simulink model "Battery"  (R2020a)
settings: Solver=FixedStepAuto  StartTime=0.0  StopTime=300  FixedStep=1e-5  RelTol=1e-3
InitFcn:
  | init;
values from neighbouring files (symbols this model uses):
  A = diag(Adiag)    [init.m]
  B = B/Cn    [init.m]
  C = eye(n)    [init.m]
  D = zeros(n,1)    [init.m]
  FCC = FCC_Ah*60*60    (= 14400)    [init.m]
  n = 4    [init.m]
  OCV = [2.8 3.4 3.6 3.7 3.8 3.9 4.0 4.1 4.2  4.4   4.6]    [init.m]
  R0 = 1.90e-3    (= 0.0019)    [init.m]
  SOC = [0    0.1    0.2  0.3 0.4   0.5   0.6  0.7  0.8    0.9 1]    [init.m]
  Ts = 0.01    [init.m]
libraries: simulink x3
settings Model: Creator=seeke  LastModifiedBy=seeke

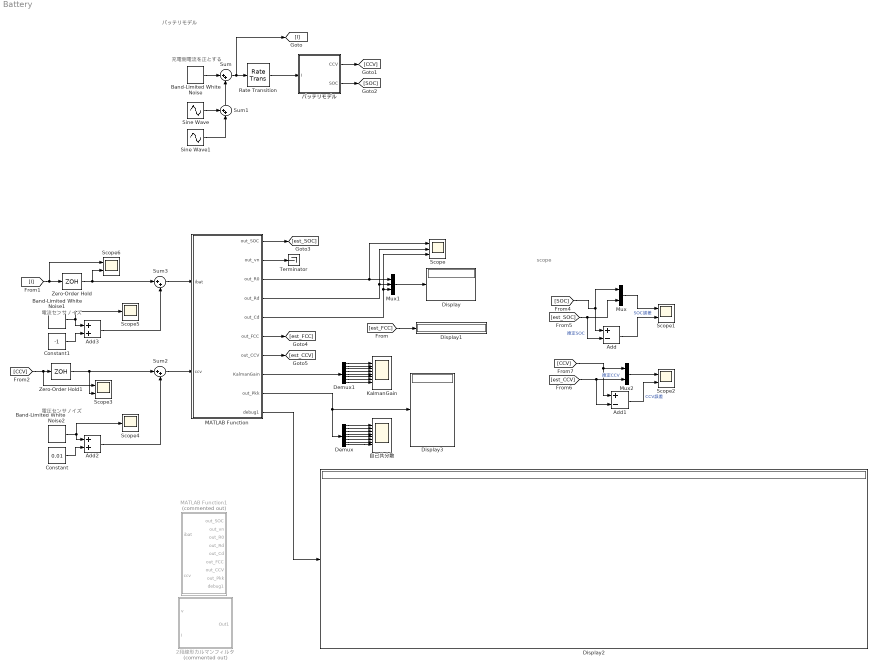
== system Battery ==
  note: 電圧センサノイズ
  note: scope
  note: バッテリモデル
  note: 充電側電流を正とする
  note: 電流センサノイズ
  2段線形カルマンフィルタ : Subsystem  Commented=on
  Add : Sum  Inputs=+-
  Add1 : Sum  Inputs=+-
  Add2 : Sum
  Add3 : Sum
  Band-Limited White Noise : simulink/Sources/Band-Limited White Noise  Cov=[100]  Ts=0.1  seed=[23341]
  Band-Limited White Noise1 : simulink/Sources/Band-Limited White Noise  Cov=[0.01]  Ts=Ts  seed=[6517]
  Band-Limited White Noise2 : simulink/Sources/Band-Limited White Noise  Cov=[0.00003]  Ts=Ts  seed=[50]
  Constant : Constant  Value=0.01
  Constant1 : Constant  Value=-1
  Demux : Demux  Outputs=8
  Demux1 : Demux  Outputs=8
  Display{,1..3} (4 alike) : Display
      Display settings: Format=short_e
      Display1 settings: Format=long_e
      Display2 settings: Format=short_e
      Display3 settings: Format=short_e
  KalmanGain : Scope  NumInputPorts=8
  MATLAB Function : MATLAB Function  TreatAsAtomicUnit=on
  MATLAB Function1 : MATLAB Function  Commented=on  TreatAsAtomicUnit=on
  Mux : Mux  Inputs=2
  Mux1 : Mux  Inputs=3
  Mux2 : Mux  Inputs=2
  Rate Transition : RateTransition
  Scope : Scope  NumInputPorts=3
  Scope{1..3,6} (4 alike) : Scope  NumInputPorts=2
  Scope4 : Scope
  Scope5 : Scope
  Sine Wave : Sin  Amplitude=100  Frequency=2*pi*0.1  SampleTime=0
  Sine Wave1 : Sin  Amplitude=30  Frequency=2*pi*0.01  SampleTime=0
  Sum : Sum  Inputs=|++
  Sum1 : Sum  Inputs=++|
  Sum2 : Sum  Inputs=|++
  Sum3 : Sum  Inputs=|++
  Terminator : Terminator
  Zero-Order Hold : ZeroOrderHold  SampleTime=Ts
  Zero-Order Hold1 : ZeroOrderHold  SampleTime=Ts
  バッテリモデル : Subsystem
  自己共分散 : Scope  NumInputPorts=8
  wires:
  Rate Transition/1 -> バッテリモデル/1(I)
  Sum/1 -> [I], Rate Transition/1
  Band-Limited White Noise/1 -> Sum/1
  バッテリモデル/1(CCV) -> [CCV]
  [CCV] -> Scope3/1, Zero-Order Hold1/1
  Zero-Order Hold1/1 -> Scope3/2, Sum2/1
  [I] -> Scope6/1, Zero-Order Hold/1
  Zero-Order Hold/1 -> Sum3/1, Scope6/2
  バッテリモデル/2(SOC) -> [SOC]
  [SOC] -> Mux/1, Add/1
  MATLAB Function/1(out_SOC) -> [est_SOC]
  MATLAB Function/6(out_FCC) -> [est_FCC]
  MATLAB Function/7(out_CCV) -> [est_CCV]
  [est_SOC] -> Mux/2, Add/2  "推定SOC"
  [CCV] -> Mux2/1, Add1/1
  [est_CCV] -> Mux2/2, Add1/2  "推定CCV"
  Add/1 -> Scope1/2  "SOC誤差"
  Mux/1 -> Scope1/1
  MATLAB Function/4(out_Rd) -> Scope/2, Mux1/2
  Mux1/1 -> Display/1
  MATLAB Function/3(out_R0) -> Scope/1, Mux1/1
  MATLAB Function/5(out_Cd) -> Scope/3, Mux1/3
  [est_FCC] -> Display1/1
  Sine Wave1/1 -> Sum1/2
  Sine Wave/1 -> Sum1/1
  Sum1/1 -> Sum/2
  MATLAB Function/10(debug1) -> Display2/1
  Mux2/1 -> Scope2/1
  Add1/1 -> Scope2/2  "CCV誤差"
  MATLAB Function/9(out_Pkk) -> Demux/1, Display3/1
  Sum2/1 -> MATLAB Function/2(ccv)
  Sum3/1 -> MATLAB Function/1(ibat)
  Add2/1 -> Sum2/2
  Constant/1 -> Add2/2
  MATLAB Function/2(out_vn) -> Terminator/1
  Constant1/1 -> Add3/2
  Add3/1 -> Sum3/2
  Band-Limited White Noise1/1 -> Scope5/1, Add3/1
  Band-Limited White Noise2/1 -> Add2/1, Scope4/1
  Demux/1 -> 自己共分散/1
  Demux/2 -> 自己共分散/2
  Demux/3 -> 自己共分散/3
  Demux/4 -> 自己共分散/4
  Demux/5 -> 自己共分散/5
  Demux/6 -> 自己共分散/6
  Demux/7 -> 自己共分散/7
  Demux/8 -> 自己共分散/8
  Demux1/8 -> KalmanGain/8
  Demux1/3 -> KalmanGain/3
  Demux1/2 -> KalmanGain/2
  Demux1/4 -> KalmanGain/4
  Demux1/7 -> KalmanGain/7
  Demux1/5 -> KalmanGain/5
  Demux1/1 -> KalmanGain/1
  MATLAB Function/8(KalmanGain) -> Demux1/1
  Demux1/6 -> KalmanGain/6

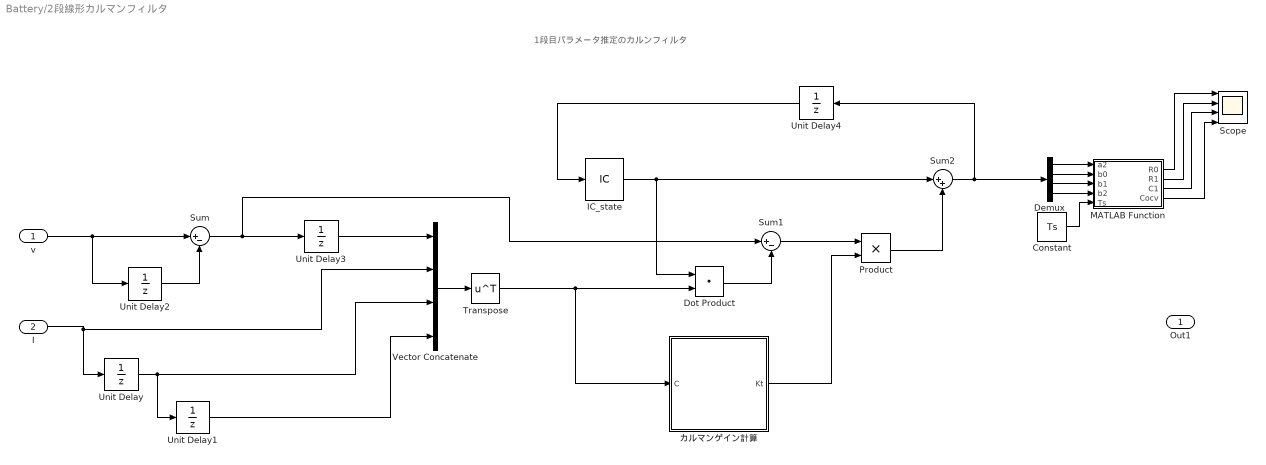
== system Battery/2段線形カルマンフィルタ ==
  note: 1段目パラメータ推定のカルンフィルタ
  v : Inport
  I : Inport  Port=2
  Constant : Constant  Value=Ts
  Demux : Demux
  Dot Product : DotProduct  InputSameDT=on  OutDataTypeStr=Inherit: Inherit via internal rule
  IC_state : InitialCondition  Value=[1 1 1 1]
  MATLAB Function : MATLAB Function  TreatAsAtomicUnit=on
  Product : Product
  Scope : Scope  NumInputPorts=4
  Sum : Sum  Inputs=|+-
  Sum1 : Sum  Inputs=|+-
  Sum2 : Sum  Inputs=|++
  Transpose : Math  Operator=transpose  SaturateOnIntegerOverflow=on
  Unit Delay{,1..4} (5 alike) : UnitDelay  SampleTime=-1  HasFrameUpgradeWarning=on
  Vector Concatenate : Concatenate  NumInputs=4  Mode=Multidimensional array
  カルマンゲイン計算 : MATLAB Function  TreatAsAtomicUnit=on
  Out1 : Outport
  wires:
  Unit Delay/1 -> Vector Concatenate/3, Unit Delay1/1
  I/1 -> Unit Delay/1, Vector Concatenate/2
  Unit Delay1/1 -> Vector Concatenate/4
  v/1 -> Unit Delay2/1, Sum/1
  Unit Delay2/1 -> Sum/2
  Sum/1 -> Sum1/1, Unit Delay3/1
  Unit Delay3/1 -> Vector Concatenate/1
  Vector Concatenate/1 -> Transpose/1
  Dot Product/1 -> Sum1/2
  Sum1/1 -> Product/1
  Product/1 -> Sum2/2
  IC_state/1 -> Sum2/1, Dot Product/1
  Transpose/1 -> Dot Product/2, カルマンゲイン計算/1(C)
  カルマンゲイン計算/1(Kt) -> Product/2
  Unit Delay4/1 -> IC_state/1
  Sum2/1 -> Unit Delay4/1, Demux/1
  Demux/1 -> MATLAB Function/1(a2)
  Demux/2 -> MATLAB Function/2(b0)
  Demux/3 -> MATLAB Function/3(b1)
  Demux/4 -> MATLAB Function/4(b2)
  Constant/1 -> MATLAB Function/5(Ts)
  MATLAB Function/1(R0) -> Scope/1
  MATLAB Function/2(R1) -> Scope/2
  MATLAB Function/3(C1) -> Scope/3
  MATLAB Function/4(Cocv) -> Scope/4

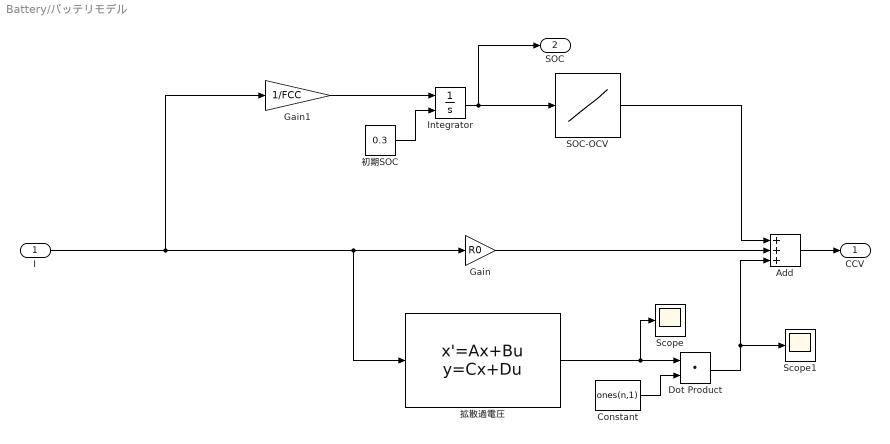
== system Battery/バッテリモデル ==
  I : Inport
  Add : Sum  Inputs=+++
  Constant : Constant  Value=ones(n,1)
  Dot Product : DotProduct  InputSameDT=on  OutDataTypeStr=Inherit: Inherit via internal rule
  Gain : Gain  Gain=R0
  Gain1 : Gain  Gain=1/FCC
  Integrator : Integrator  InitialConditionSource=external
  SOC-OCV : Lookup_n-D  NumberOfTableDimensions=1  BreakpointsForDimension1=SOC  Table=OCV  InternalRulePriority=Speed  RndMeth=Simplest  InputSameDT=on
  Scope : Scope
  Scope1 : Scope
  初期SOC : Constant  Value=0.3
  拡散過電圧 : StateSpace  A=A  B=B  C=C  D=D  InitialCondition=0
  CCV : Outport
  SOC : Outport  Port=2
  wires:
  拡散過電圧/1 -> Scope/1, Dot Product/1
  Gain/1 -> Add/2
  I/1 -> 拡散過電圧/1, Gain/1, Gain1/1
  SOC-OCV/1 -> Add/1
  初期SOC/1 -> Integrator/2
  Constant/1 -> Dot Product/2
  Dot Product/1 -> Add/3, Scope1/1
  Gain1/1 -> Integrator/1
  Integrator/1 -> SOC/1, SOC-OCV/1
  Add/1 -> CCV/1

== matlab function Battery/2段線形カルマンフィルタ/カルマンゲイン計算 ==
  data: Kt output; C input
function Kt = fcn(C)

%Qt  = diag([1 1 1 1]);       %[m×m]プロセス白色雑音wの分散
Qt = 0.1;
Gt = [0.1; 0.1; 0.1; 0.1];                   %[n×m]プロセス白色雑音wの係数 Gt*w

R = 1;                                 %観測雑音の共分散

persistent est_theta P 
if isempty(est_theta)
    est_theta = [1; 1; 1; 1];                   %推定値の初期値
    P = diag([0.1 0.1 0.1 0.1]);                          %状態の事前分布の共分散行列
end

%% 観測更新ステップ
%カルマンゲインの計算
Kt = P*C.'*[C * P * C.' + R]^-1;

%フィルタ推定値
%est_theta = est_theta + Kt*(y - C*est_theta);

%推定誤差共分散行列
 P = P - Kt*C*P;

 %% 時間更新ステップ
 %1段予測推定値
 %est_theta = 1*est_theta ;
 
 %予測誤差共分散行列
 P = 1*P*1 + Gt*Qt*Gt.';

== matlab function Battery/MATLAB Function1 ==
  data: ibat input; ccv input; out_SOC output; out_vn output; out_R0 output; out_Rd output; out_Cd output; out_FCC output; out_CCV output; out_Pkk output; debug1 output
function [out_SOC,out_vn,out_R0,out_Rd,out_Cd,out_FCC, out_CCV,out_Pkk,debug1] = ukf(ibat,ccv)

Ts = 0.01;       %[s]サンプル時間
n = 3;             %拡散項の等価回路近似次数
nz = (n +1) +4;                %状態変数zの次元 x の次数がn+1、thetaの次数が4
lambda = 3 + nz;        %論文だと3-nzなんだけど…

% gamma =sqrt(nz+lambda);         %シグマポイントの推定中心からのずらす量重み
gamma = 0.4; 

r = 0.01;       % 観測雑音の分散

%システム雑音の自己共分散を決める
Q_SOC = 10e-3;
Q_v      = ones(1,n)*10e-4;         %拡散項の過電圧のシステム雑音
Q_R0    = 10e-3;
Q_Rd    = 10e-3;
Q_Cd     = 10e-2;
Q_FCC    = 10;
Q = diag( [Q_SOC Q_v Q_R0 Q_Rd Q_Cd Q_FCC] );         %システム雑音

%永続変数の定義、次のループでも持っておかないといけない値
%初期化
persistent est_zkk Skk
if isempty(est_zkk)
%      est_zkk = [0.3 ; ones(n,1)*0; log(1.90e-3); log(1.42e-3); log(1.65e5); log(13000)];   %%拡大系の状態変数、z = [x;theta]推定値の初期化   
    est_zkk = [0.4 ; ones(n,1)*0; log(1.00e-3); log(0.5e-3); log(1.0e5); log(13000)];
    Skk        =  diag([0.1, ones(1,n)*0.5, log(10e-3), log(10e-3), log(5000), log(4000)]);   %拡大系の自己共分散の平方根行列
end

alpha = 1;
beta   = 2;

wm = [lambda/(nz+lambda); ones(2*nz,1)*1/2/(nz+lambda)];    %平均値に対するシグマポイントの重み
wc  = [(lambda/(nz+lambda))+1-alpha^2+beta; ones(2*nz,1)*1/2/(nz+lambda)];      %共分散に対するシグマポイントの重み

%事前推定

%シグマポイントの生成
Zkk = zeros(nz,2*nz+1);     %シグマポイント初期化
Zkk(:,1) = est_zkk;                                                                     %i=0代入
Zkk(:,2:nz+1) = repmat(est_zkk,1,nz) + gamma*Skk;             %i=1～nz
Zkk(:,nz+2:2*nz+1) = repmat(est_zkk,1,nz) - gamma*Skk;   %i=nz+1～2nz

%シグマポイントごとに状態方程式を用いて事前推定を行う
Zk1k = zeros(nz,2*nz+1);     %シグマポイント初期化
est_zk1k =  zeros(nz,1);    %k+1|kの状態変数推定値を初期化
for i = 1:2*nz+1
    %シグマポイントの更新
    Zk1k(:,i) =  fd(Zkk(:,i),ibat,n,Ts);

   %重みをかけながら、シグマポイントの平均を求める
    est_zk1k = est_zk1k + wm(i,1)*Zk1k(:,i);
end

if  wc(1)>=0      %重みが正のときはQR分解
    Mk1k  = zeros(nz,2*nz+1);    %誤差共分散の平方根行列の初期化
else
    Mk1k  = zeros(nz,2*nz);    %誤差共分散の平方根行列の初期化
end

%誤差共分散行列の平方根行列を求める
if  wc(1)>=0      %重みが正のときはQR分解
    for i = 1:2*nz+1
        %誤差共分散の平方根行列をシグマポイントを使って計算
        Mk1k(:,i) = sqrt(wc(i))* (Zk1k(:,i)-est_zk1k);
    end    
    qr_Sk1k = qr([Mk1k sqrt(Q)]');
    Sk1k = qr_Sk1k(1:nz,1:nz);
    
else            %重みの項はQR分解使えないので、コレスキー分解の1ランク更新を組み合わせて使う
    for i = 1:2*nz
        %誤差共分散の平方根行列をシグマポイントを使って計算
        Mk1k(:,i) = sqrt(wc(i))* (Zk1k(:,i)-est_zk1k);
    end
    Tk1k = qr([Mk1k sqrt(Q)]);         %正定でQR分解できるところ
    Sk1k = cholupdate(Tk1k,sqrt(wc(1)*(Zk1k(:,1)-est_zk1k)),'-');   %コレスキー分解のdowndate
    
end

%事前推定値zk1kを用いてシグマポイントを再生成
Zk1k(:,1) = est_zk1k;
Zk1k(:,2:nz+1) =  repmat(est_zk1k,1,nz) + gamma*Sk1k;
Zk1k(:,nz+2:2*nz+1) =  repmat(est_zk1k,1,nz) -  gamma*Sk1k;

%出力方程式から事前推定
est_yk1k = 0;                           %初期化
Yk1k = zeros(1,2*nz+1);       %初期化
for i = 1:2*nz+1
    Yk1k(1,i) = hd(Zk1k(:,i),ibat,n);                    %シグマポイントごとに出力のポイントも生成    
    est_yk1k = est_yk1k +  wm(i)*Yk1k(1,i);    %重みを使って、出力の推定値を計算
end

%k+1|kの誤差の共分散行列を更新する
Mzz_k1k = zeros(nz,2*nz+1);      %初期化
Myy_k1k = zeros(1,2*nz+1);        %初期化
if wc(1)>=0     %重みが正のときはQR分解で計算する
    for i = 1:2*nz+1
        Mzz_k1k(:,i) = sqrt(wc(i))*(Zk1k(:,i) -est_zk1k);
        Myy_k1k(:,i) = sqrt(wc(i))*(Yk1k(1,i)-est_yk1k);
    end
    Syy_k1k = qr([Myy_k1k sqrt(r)]);
    Pzy_k1k = Mzz_k1k*(Myy_k1k)';
else    %重みが負であるときはQR分解とコレスキー分解のランク1更新を組み合わせて使う
    
    %とりあえず重み負にならない設定で運用
    %
    
end

%事後推定
Kk1k = Pzy_k1k/(Syy_k1k*Syy_k1k');
est_zk1k1= est_zk1k + Kk1k*(ccv - est_yk1k);
Sk1k1 = qr([Mzz_k1k - (Kk1k*Myy_k1k) , sqrt(r)*Kk1k]');

debug1 = Sk1k1 ;

%次回のループ用に更新
est_zkk = est_zk1k1;
Skk = Sk1k1(1:nz,1:nz);



% 出力の設定
out_SOC  = est_zk1k1(1,1);
out_vn     = exp(est_zk1k1(2:1+n,1));
out_R0   =  exp(est_zk1k1(end-3,1));
out_Rd   = exp(est_zk1k1(end-2,1));
out_Cd   = exp(est_zk1k1(end-1,1));
out_FCC = exp(est_zk1k1(end,1));

out_CCV =est_yk1k;

out_Pkk = diag(Skk'*Skk);    %自己共分散行列

% out_Pkk = Skk;
% [Skk(:,1);Skk(:,2)]; 

end

%********以下、状態方程式とかmain外の関数**********************

%%  連続時間で定義した状態方式
%n拡散項の 過電圧の次元
%現時刻の状態変数z
%入力u
%theta = [lnR0 ; lnRd ; lnCd ; lnFCC]　対数化したパラメータ
function dzk = fl(zk,ik,n)
%引数をばらす
nz = n + 5;  %zの次元
aR0 = zk(nz-3);     %パラメータは後半の4つ分
aRd = zk(nz-2);
aCd = zk(nz-1);
aFCC = zk(nz);
vk = zk(2:n+1);         %拡散による過電圧

%配列確保しておく
dzk = zeros(nz,1);      %列ベクトルとして確保

%更新
dzk(1,1) = ik/exp(aFCC);    %SOC

for j = 1:n
    dzk(j+1,1) = -(2*j-1)^2*pi^2*vk(j)/4/exp(aCd+aRd)+2*ik/exp(aCd);    %過電圧
end

%パラメータ
dzk(nz-3,1) = 0;        %aR0
dzk(nz-2,1) = 0;        %aRd
dzk(nz-1,1) = 0;        %aCd
dzk(nz,1) = 0;        %aFCC

end

%% ルンゲクッタ法で時刻の更新を行う
%n 拡散項の近似次数
%Ts サンプル時間
function zk1 = fd(zk,ik,n,Ts)

c1 = fl(zk,ik,n);
c2 = fl(zk+Ts/2*c1,ik,n);
c3 = fl(zk+Ts/2*c2,ik,n);
c4 = fl(zk+Ts*c3,ik,n);

zk1 = zk + Ts/6 *(c1+2*c2+2*c3+c4);

end


%% 出力方程式
%n　拡散項の近似次数
function  CCVk = hd(zk,ik,n)

SOC = [0    0.1    0.2  0.3 0.4   0.5   0.6  0.7  0.8    0.9 1];
OCV = [2.8 3.4 3.6 3.7 3.8 3.9 4.0 4.1 4.2  4.4   4.6];

%OCV
CCVk = interp1(SOC,OCV,zk(1,1));

%拡散項の過電圧
for i=1:n
    CCVk = CCVk + zk(1+i);
end
    
%R0による部分
CCVk = CCVk + exp(zk(end-3))*ik;

end

== matlab function Battery/2段線形カルマンフィルタ/MATLAB Function ==
  data: a2 input; R0 output; b0 input; b1 input; b2 input; R1 output; C1 output; Cocv output; Ts input
function [R0,R1,C1,Cocv ] = fcn(a2, b0, b1, b2, Ts)

R0 = b0;

R1 = - (a2^2 +a2*b1 +b2)/(1-a2)^2;

C1 = -Ts*(1-a2)/(a2^2*b0+a2*b1+b2);

Cocv = Ts * (1-a2)/(b0+b1+b2);

== matlab function Battery/MATLAB Function ==
  data: ibat input; ccv input; out_SOC output; out_vn output; out_R0 output; out_Rd output; out_Cd output; out_FCC output; out_CCV output; KalmanGain output; out_Pkk output; debug1 output
function [out_SOC,out_vn,out_R0,out_Rd,out_Cd,out_FCC, out_CCV,KalmanGain,out_Pkk,debug1] = ukf(ibat,ccv)

Ts = 0.01;       %[s]サンプル時間
n = 3;             %拡散項の等価回路近似次数
nz = (n +1) +4;                %状態変数zの次元 x の次数がn+1、thetaの次数が4
lambda = 3 + nz;        %論文だと3-nzなんだけど…

% gamma =sqrt(nz+lambda);         %シグマポイントの推定中心からのずらす量重み
gamma = 0.6;

r = 0.01;       % 観測雑音の分散

%システム雑音の自己共分散を決める
Q_SOC = 10e-4;
Q_v      = ones(1,n)*10e-4;         %拡散項の過電圧のシステム雑音
Q_R0   = 1e-3;
Q_Rd   = 1e-5;
Q_Cd    = 1e-4;
Q_FCC  = 1e-2;
Q = diag( [Q_SOC Q_v Q_R0 Q_Rd Q_Cd Q_FCC] );         %システム雑音

%永続変数の定義、次のループでも持っておかないといけない値
%初期化
persistent est_zkk Skk
if isempty(est_zkk)
%      est_zkk = [0.3 ; ones(n,1)*0; log(1.90e-3); log(1.42e-3); log(1.65e5); log(14400)];   %%拡大系の状態変数、z = [x;theta]推定値の初期化   
    est_zkk = [0.38 ; ones(n,1)*0; log(1.00e-3); log(0.5e-3); log(1.3e5); log(13000)];
    Skk        =  diag([0.1, ones(1,n)*0.5, log(10e-1), log(10e-1), log(5000), log(5000)]);   %拡大系の自己共分散の平方根行列
end

alpha = 1;
beta   = 2;

wm = [lambda/(nz+lambda); ones(2*nz,1)*1/2/(nz+lambda)];    %平均値に対するシグマポイントの重み
wc  = [(lambda/(nz+lambda))+1-alpha^2+beta; ones(2*nz,1)*1/2/(nz+lambda)];      %共分散に対するシグマポイントの重み

%事前推定*************************

%シグマポイントの生成
Zkk = zeros(nz,2*nz+1);     %シグマポイント初期化
Zkk(:,1) = est_zkk;                                                                     %i=0代入
Zkk(:,2:nz+1)            = repmat(est_zkk,1,nz) + gamma*Skk;             %i=1～nz
Zkk(:,nz+2:2*nz+1) = repmat(est_zkk,1,nz) - gamma*Skk;   %i=nz+1～2nz

%シグマポイントごとに状態方程式を用いて事前推定を行う
Zk1k = zeros(nz,2*nz+1);     %シグマポイント初期化
est_zk1k =  zeros(nz,1);    %k+1|kの状態変数推定値を初期化
for i = 1:2*nz+1
    
    Zk1k(:,i) =  fd(Zkk(:,i),ibat,n,Ts);    %シグマポイントの更新

    est_zk1k = est_zk1k + wm(i)*Zk1k(:,i);  %重みをかけながら、シグマポイントの平均を求める
end

if  wc(1)>=0      %重みが正のときはQR分解
    Mk1k  = zeros(nz,2*nz+1);    %誤差共分散の平方根行列の初期化
else
    Mk1k  = zeros(nz,2*nz);    %誤差共分散の平方根行列の初期化
end

%誤差共分散行列の平方根行列を求める
if  wc(1)>=0      %重みが正のときはQR分解
    for i = 1:2*nz+1
        Mk1k(:,i) = sqrt(wc(i))*(Zk1k(:,i)-est_zk1k);   %誤差共分散の平方根行列をシグマポイントを使って計算
    end    
    
    [qrQ_Sk1k, qrR_Sk1k] = qr([Mk1k ,sqrt(Q)]');
    Sk1k = qrR_Sk1k(1:nz,1:nz);
    
else            %重みの項はQR分解使えないので、コレスキー分解の1ランク更新を組み合わせて使う
    for i = 1:2*nz
        %誤差共分散の平方根行列をシグマポイントを使って計算
        Mk1k(:,i) = sqrt(wc(i))* (Zk1k(:,i)-est_zk1k);
    end
    Tk1k = qr([Mk1k sqrt(Q)]);         %正定でQR分解できるところ
    Sk1k = cholupdate(Tk1k,sqrt(wc(1)*(Zk1k(:,1)-est_zk1k)),'-');   %コレスキー分解のdowndate

end

%事前推定値zk1kを用いてシグマポイントを再生成
Zk1k(:,1) = est_zk1k;
Zk1k(:,2:nz+1) =  repmat(est_zk1k,1,nz) + gamma*Sk1k;
Zk1k(:,nz+2:2*nz+1) =  repmat(est_zk1k,1,nz) -  gamma*Sk1k;

%出力方程式から事前推定
est_yk1k = 0;                           %初期化
Yk1k = zeros(1,2*nz+1);       %初期化
for i = 1:2*nz+1
    Yk1k(1,i) = hd(Zk1k(:,i),ibat,n);                    %シグマポイントごとに出力のポイントも生成    
    est_yk1k = est_yk1k +  wm(i)*Yk1k(1,i);    %重みを使って、出力の推定値を計算
end

%k+1|kの誤差の共分散行列を更新する
Mzz_k1k = zeros(nz,2*nz+1);      %初期化
Myy_k1k = zeros(1,2*nz+1);        %初期化
if wc(1)>=0     %重みが正のときはQR分解で計算する
    for i = 1:2*nz+1
        Mzz_k1k(:,i) = sqrt(wc(i))*(Zk1k(:,i) -est_zk1k);
        Myy_k1k(:,i) = sqrt(wc(i))*(Yk1k(1,i)-est_yk1k);
    end
    [qrQ_Syy_k1k,qrR_Syy_k1k] = qr([Myy_k1k ,sqrt(r)]');
    Syy_k1k = qrR_Syy_k1k;
    Pzy_k1k = Mzz_k1k*(Myy_k1k)';
    
    debug1 =  Myy_k1k;
    
else    %重みが負であるときはQR分解とコレスキー分解のランク1更新を組み合わせて使う
    
    %とりあえず重み負にならない設定で運用
    %
    
end

%事後推定
Kk1k = Pzy_k1k/(Syy_k1k'*Syy_k1k);                  %カルマンゲインの計算

est_zk1k1= est_zk1k + Kk1k*(ccv - est_yk1k);    %イノベーション過程
[qrQ_Sk1k1, qrR_Sk1k1]= qr([Mzz_k1k - (Myy_k1k'*Kk1k')' , sqrt(r)*Kk1k]');
Sk1k1 = qrR_Sk1k1;

% debug1 = est_zk1k1 ;

%次回のループ用に更新
est_zkk = est_zk1k1;
Skk = Sk1k1(1:nz,1:nz);

% 出力の設定
out_SOC = est_zk1k1(1,1);
out_vn    = exp(est_zk1k1(2:1+n,1));
out_R0   =  exp(est_zk1k1(end-3,1));
out_Rd   = exp(est_zk1k1(end-2,1));
out_Cd   = exp(est_zk1k1(end-1,1));
out_FCC = exp(est_zk1k1(end,1));
KalmanGain=Kk1k;
out_CCV =est_yk1k;
out_Pkk = diag(Skk'*Skk);    %自己共分散行列

end

%***********************以下、状態方程式とかmain外の関数***************************







%%  連続時間で定義した状態方式
%n拡散項の 過電圧の次元
%現時刻の状態変数z
%入力u
%theta = [lnR0 ; lnRd ; lnCd ; lnFCC]　対数化したパラメータ
function dzk = fl(zk,ik,n)
%引数をばらす
nz = n + 5;  %zの次元
aR0 = zk(nz-3);     %パラメータは後半の4つ分
aRd = zk(nz-2);
aCd = zk(nz-1);
aFCC = zk(nz);
vk = zk(2:n+1);         %拡散による過電圧

%配列確保しておく
dzk = zeros(nz,1);      %列ベクトルとして確保

%更新
dzk(1,1) = ik/exp(aFCC);    %SOC

for j = 1:n
    dzk(j+1,1) = -(2*j-1)^2*pi^2*vk(j)/4/exp(aCd+aRd)+2*ik/exp(aCd);    %過電圧
end

%パラメータ
dzk(nz-3,1) = 0;        %aR0
dzk(nz-2,1) = 0;        %aRd
dzk(nz-1,1) = 0;        %aCd
dzk(nz,1) = 0;        %aFCC

end

%% ルンゲクッタ法で時刻の更新を行う
%n 拡散項の近似次数
%Ts サンプル時間
function zk1 = fd(zk,ik,n,Ts)

c1 = fl(zk,ik,n);
c2 = fl(zk+Ts/2*c1,ik,n);
c3 = fl(zk+Ts/2*c2,ik,n);
c4 = fl(zk+Ts*c3,ik,n);

zk1 = zk + Ts/6 *(c1+2*c2+2*c3+c4);

end


%% 出力方程式
%n　拡散項の近似次数
function  CCVk = hd(zk,ik,n)

SOC = [0    0.1    0.2  0.3 0.4   0.5   0.6  0.7  0.8    0.9 1];
OCV = [2.8 3.4 3.6 3.7 3.8 3.9 4.0 4.1 4.2  4.4   4.6];

%OCV
CCVk = interp1(SOC,OCV,zk(1,1));

%拡散項の過電圧
for i=1:n
    CCVk = CCVk + zk(1+i);
end
    
%R0による部分
CCVk = CCVk + exp(zk(end-3))*ik;

end
